simulink model "ev13_registros"  (R2023b)
settings: Solver=VariableStepAuto  StartTime=0.0  StopTime=inf  RelTol=1e-3
libraries: simulink_extras x10
settings Model: Creator=juanm  LastModifiedBy=juanm

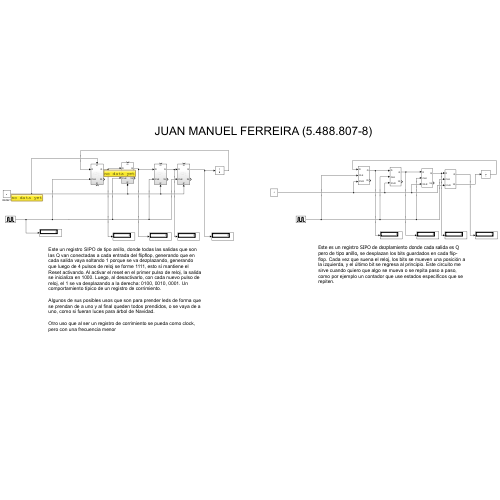
[thumbnail: Simulink's stored preview of the top-level diagram]
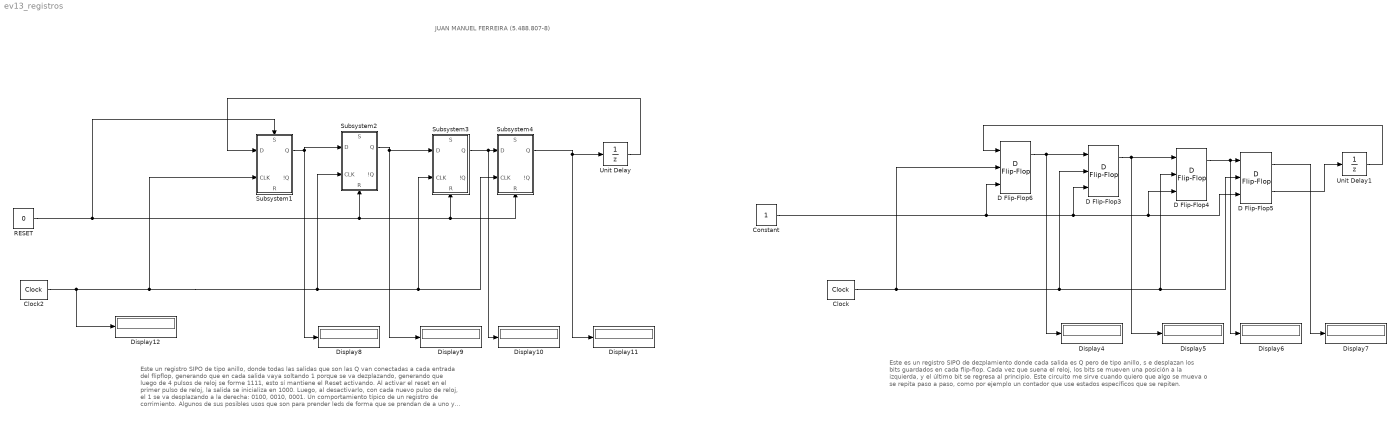
== system ev13_registros ==
  note: JUAN MANUEL FERREIRA (5.488.807-8)
  note: Este es un registro SIPO de dezplamiento donde cada salida es Q pero de tipo anillo, s e desplazan los bits guardados en cada flip-flop. Cada vez que suena el reloj, los bits se mueven una posición a la izquierda, y el último bit se regresa al principio. Este circuito me sirve cuando quiero que algo se mueva o se repita paso a paso, como por ejemplo un contador que use estados específicos que se repiten.
  note: Este un registro SIPO de tipo anillo, donde todas las salidas que son las Q van conectadas a cada entrada del flipflop, generando que en cada salida vaya soltando 1 porque se va dezplazando, generando que luego de 4 pulsos de reloj se forme 1111, esto sí mantiene el Reset activando. Al activar el reset en el primer pulso de reloj, la salida se inicializa en 1000. Luego, al desactivarlo, con cada nuevo pulso de reloj, el 1 se va desplazando a la derecha: 0100, 0010, 0001. Un comportamiento típico de un registro de corrimiento.
      |
      | Algunos de sus posibles usos que son para prender leds de forma que se prendan de a uno y al final queden todos prendidos, o se vaya de a uno, como si fueran luces para árbol de Navidad.
      |
      | Otro uso que al ser un registro de corrimiento se pueda como clock, pero con una frecuencia menor
  Clock : simulink_extras/Flip Flops/Clock  period=2
  Clock2 : simulink_extras/Flip Flops/Clock  period=2
  Constant : Constant
  D Flip-Flop{3..6} (4 alike) : simulink_extras/Flip Flops/D Flip-Flop
  Display{4..12} (9 alike) : Display
  RESET : Constant  Value=0  OutDataTypeStr=boolean
  Subsystem1 : Subsystem
      settings: PortSchema="{\"entries\":[{\"content\":{\"sides\":[{\"content\":{\"connectorIds\":[\"In1\",\"In2\"]},\"type\":\"ConnectorPlacement.EquallySpacedRectSide\",\"uuid\":\"e3878c95-46f3-4509-9baa-e715f418dba1\"},{\"content\":{\"connectorIds\":[\"Out1\",\"Out2\"],\"side\":\"RIGHT\"},\"type\":\"ConnectorPlacement.EquallySpacedRectSide\",\"uuid\":\"07877722-e247-4eb2-8428-8296816940c1\"},{\"content\":{\"connectorIds\":[\"In3\"],\"side\":\"TOP\"},\"type\":\"ConnectorPlacement.EquallySpacedRectSide\",\"uuid\":\"8cc11adc-8fe2-4fc3-91be-12b2d4a599d3\"},{\"content\":{\"connectorIds\":[\"In4\"],\"side\":\"BOTTOM\"},\"type\":\"ConnectorPlacement.EquallySpacedRectSide\",\"uuid\":\"07da6bee-c4ce-4432-ad6f-4d7b93f4049b\"}]},\"type\":\"ConnectorPlacement.EquallySpacedConnector\",\"uuid\":\"c12c8677-41de-4e24-9f13-5794546de7c9\"}],\"packageUris\":[\"http://schema.mathworks.com/mf0/Connector/R2020b\"],\"version\":\"1.0\"}"
  Subsystem2 : Subsystem
      settings: PortSchema="{\"entries\":[{\"content\":{\"sides\":[{\"content\":{\"connectorIds\":[\"In1\",\"In2\"]},\"type\":\"ConnectorPlacement.EquallySpacedRectSide\",\"uuid\":\"e3878c95-46f3-4509-9baa-e715f418dba1\"},{\"content\":{\"connectorIds\":[\"Out1\",\"Out2\"],\"side\":\"RIGHT\"},\"type\":\"ConnectorPlacement.EquallySpacedRectSide\",\"uuid\":\"07877722-e247-4eb2-8428-8296816940c1\"},{\"content\":{\"connectorIds\":[\"In3\"],\"side\":\"TOP\"},\"type\":\"ConnectorPlacement.EquallySpacedRectSide\",\"uuid\":\"8cc11adc-8fe2-4fc3-91be-12b2d4a599d3\"},{\"content\":{\"connectorIds\":[\"In4\"],\"side\":\"BOTTOM\"},\"type\":\"ConnectorPlacement.EquallySpacedRectSide\",\"uuid\":\"07da6bee-c4ce-4432-ad6f-4d7b93f4049b\"}]},\"type\":\"ConnectorPlacement.EquallySpacedConnector\",\"uuid\":\"c12c8677-41de-4e24-9f13-5794546de7c9\"}],\"packageUris\":[\"http://schema.mathworks.com/mf0/Connector/R2020b\"],\"version\":\"1.0\"}"
  Subsystem3 : Subsystem
      settings: PortSchema="{\"entries\":[{\"content\":{\"sides\":[{\"content\":{\"connectorIds\":[\"In1\",\"In2\"]},\"type\":\"ConnectorPlacement.EquallySpacedRectSide\",\"uuid\":\"e3878c95-46f3-4509-9baa-e715f418dba1\"},{\"content\":{\"connectorIds\":[\"Out1\",\"Out2\"],\"side\":\"RIGHT\"},\"type\":\"ConnectorPlacement.EquallySpacedRectSide\",\"uuid\":\"07877722-e247-4eb2-8428-8296816940c1\"},{\"content\":{\"connectorIds\":[\"In3\"],\"side\":\"TOP\"},\"type\":\"ConnectorPlacement.EquallySpacedRectSide\",\"uuid\":\"8cc11adc-8fe2-4fc3-91be-12b2d4a599d3\"},{\"content\":{\"connectorIds\":[\"In4\"],\"side\":\"BOTTOM\"},\"type\":\"ConnectorPlacement.EquallySpacedRectSide\",\"uuid\":\"07da6bee-c4ce-4432-ad6f-4d7b93f4049b\"}]},\"type\":\"ConnectorPlacement.EquallySpacedConnector\",\"uuid\":\"c12c8677-41de-4e24-9f13-5794546de7c9\"}],\"packageUris\":[\"http://schema.mathworks.com/mf0/Connector/R2020b\"],\"version\":\"1.0\"}"
  Subsystem4 : Subsystem
      settings: PortSchema="{\"entries\":[{\"content\":{\"sides\":[{\"content\":{\"connectorIds\":[\"In1\",\"In2\"]},\"type\":\"ConnectorPlacement.EquallySpacedRectSide\",\"uuid\":\"e3878c95-46f3-4509-9baa-e715f418dba1\"},{\"content\":{\"connectorIds\":[\"Out1\",\"Out2\"],\"side\":\"RIGHT\"},\"type\":\"ConnectorPlacement.EquallySpacedRectSide\",\"uuid\":\"07877722-e247-4eb2-8428-8296816940c1\"},{\"content\":{\"connectorIds\":[\"In3\"],\"side\":\"TOP\"},\"type\":\"ConnectorPlacement.EquallySpacedRectSide\",\"uuid\":\"8cc11adc-8fe2-4fc3-91be-12b2d4a599d3\"},{\"content\":{\"connectorIds\":[\"In4\"],\"side\":\"BOTTOM\"},\"type\":\"ConnectorPlacement.EquallySpacedRectSide\",\"uuid\":\"07da6bee-c4ce-4432-ad6f-4d7b93f4049b\"}]},\"type\":\"ConnectorPlacement.EquallySpacedConnector\",\"uuid\":\"c12c8677-41de-4e24-9f13-5794546de7c9\"}],\"packageUris\":[\"http://schema.mathworks.com/mf0/Connector/R2020b\"],\"version\":\"1.0\"}"
  Unit Delay : UnitDelay  SampleTime=-1  HasFrameUpgradeWarning=on
  Unit Delay1 : UnitDelay  SampleTime=-1  HasFrameUpgradeWarning=on
  wires:
  D Flip-Flop3/1 -> D Flip-Flop4/1, Display5/1
  D Flip-Flop4/1 -> D Flip-Flop5/1, Display6/1
  Unit Delay1/1 -> D Flip-Flop6/1
  D Flip-Flop6/1 -> D Flip-Flop3/1, Display4/1
  Clock/1 -> D Flip-Flop3/2, D Flip-Flop4/2, D Flip-Flop5/2, D Flip-Flop6/2
  Constant/1 -> D Flip-Flop6/3, D Flip-Flop3/3, D Flip-Flop4/3, D Flip-Flop5/3
  D Flip-Flop5/2 -> Unit Delay1/1
  D Flip-Flop5/1 -> Display7/1
  Subsystem2/1(Q) -> Subsystem3/1(D), Display9/1
  Subsystem3/1(Q) -> Subsystem4/1(D), Display10/1
  Subsystem4/1(Q) -> Display11/1, Unit Delay/1
  Subsystem1/1(Q) -> Subsystem2/1(D), Display8/1
  Clock2/1 -> Display12/1, Subsystem1/2(CLK), Subsystem2/2(CLK), Subsystem3/2(CLK), Subsystem4/2(CLK)
  RESET/1 -> Subsystem2/4(R), Subsystem3/4(R), Subsystem4/4(R), Subsystem1/3(S)
  Unit Delay/1 -> Subsystem1/1(D)

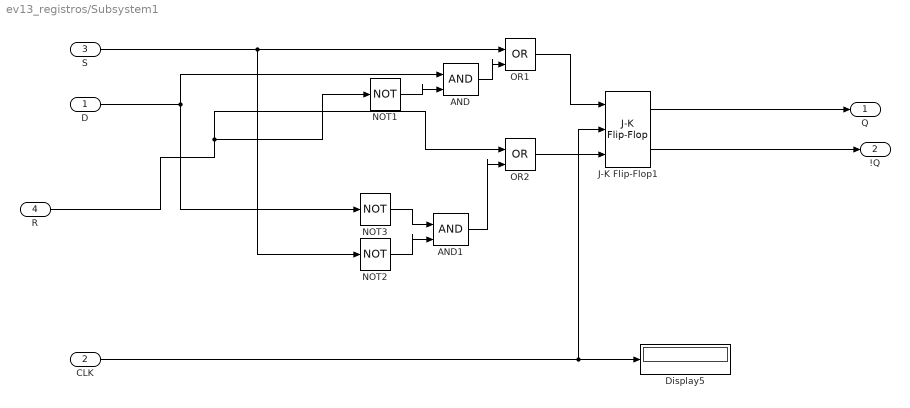
== system ev13_registros/Subsystem1 ==
  D : Inport
  CLK : Inport  Port=2
  S : Inport  Port=3
  R : Inport  Port=4
  AND : Logic  IconShape=distinctive  AllPortsSameDT=off  OutDataTypeStr=boolean
  AND1 : Logic  IconShape=distinctive  AllPortsSameDT=off  OutDataTypeStr=boolean
  Display5 : Display
  J-K Flip-Flop1 : simulink_extras/Flip Flops/J-K Flip-Flop  initial_condition=0
  NOT1 : Logic  Operator=NOT  IconShape=distinctive  AllPortsSameDT=off  OutDataTypeStr=boolean
  NOT2 : Logic  Operator=NOT  IconShape=distinctive  AllPortsSameDT=off  OutDataTypeStr=boolean
  NOT3 : Logic  Operator=NOT  IconShape=distinctive  AllPortsSameDT=off  OutDataTypeStr=boolean
  OR1 : Logic  Operator=OR  IconShape=distinctive  AllPortsSameDT=off  OutDataTypeStr=boolean
  OR2 : Logic  Operator=OR  IconShape=distinctive  AllPortsSameDT=off  OutDataTypeStr=boolean
  Q : Outport
  !Q : Outport  Port=2
  wires:
  R/1 -> NOT1/1, OR2/1
  S/1 -> OR1/1, NOT2/1
  J-K Flip-Flop1/1 -> Q/1
  AND/1 -> OR1/2
  NOT2/1 -> AND1/2
  NOT1/1 -> AND/2
  OR2/1 -> J-K Flip-Flop1/3
  CLK/1 -> Display5/1, J-K Flip-Flop1/2
  AND1/1 -> OR2/2
  J-K Flip-Flop1/2 -> !Q/1
  OR1/1 -> J-K Flip-Flop1/1
  NOT3/1 -> AND1/1
  D/1 -> AND/1, NOT3/1

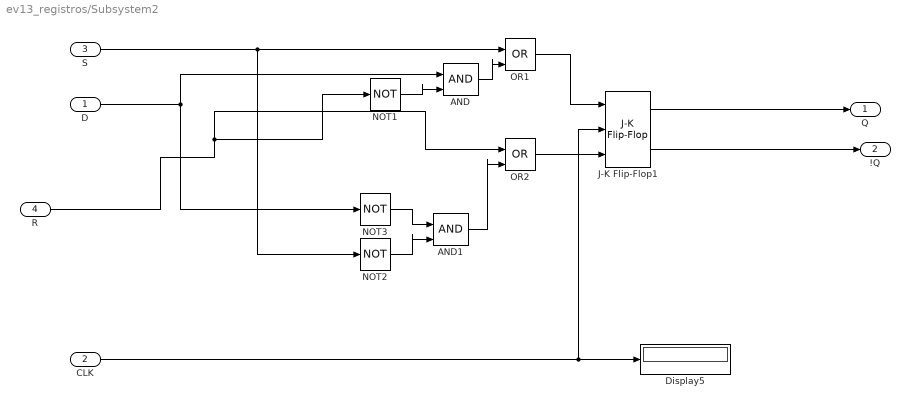
== system ev13_registros/Subsystem2 ==
  D : Inport
  CLK : Inport  Port=2
  S : Inport  Port=3
  R : Inport  Port=4
  AND : Logic  IconShape=distinctive  AllPortsSameDT=off  OutDataTypeStr=boolean
  AND1 : Logic  IconShape=distinctive  AllPortsSameDT=off  OutDataTypeStr=boolean
  Display5 : Display
  J-K Flip-Flop1 : simulink_extras/Flip Flops/J-K Flip-Flop  initial_condition=0
  NOT1 : Logic  Operator=NOT  IconShape=distinctive  AllPortsSameDT=off  OutDataTypeStr=boolean
  NOT2 : Logic  Operator=NOT  IconShape=distinctive  AllPortsSameDT=off  OutDataTypeStr=boolean
  NOT3 : Logic  Operator=NOT  IconShape=distinctive  AllPortsSameDT=off  OutDataTypeStr=boolean
  OR1 : Logic  Operator=OR  IconShape=distinctive  AllPortsSameDT=off  OutDataTypeStr=boolean
  OR2 : Logic  Operator=OR  IconShape=distinctive  AllPortsSameDT=off  OutDataTypeStr=boolean
  Q : Outport
  !Q : Outport  Port=2
  wires:
  D/1 -> NOT3/1, AND/1
  NOT3/1 -> AND1/1
  OR1/1 -> J-K Flip-Flop1/1
  J-K Flip-Flop1/2 -> !Q/1
  AND1/1 -> OR2/2
  CLK/1 -> J-K Flip-Flop1/2, Display5/1
  OR2/1 -> J-K Flip-Flop1/3
  NOT1/1 -> AND/2
  NOT2/1 -> AND1/2
  AND/1 -> OR1/2
  J-K Flip-Flop1/1 -> Q/1
  S/1 -> NOT2/1, OR1/1
  R/1 -> OR2/1, NOT1/1

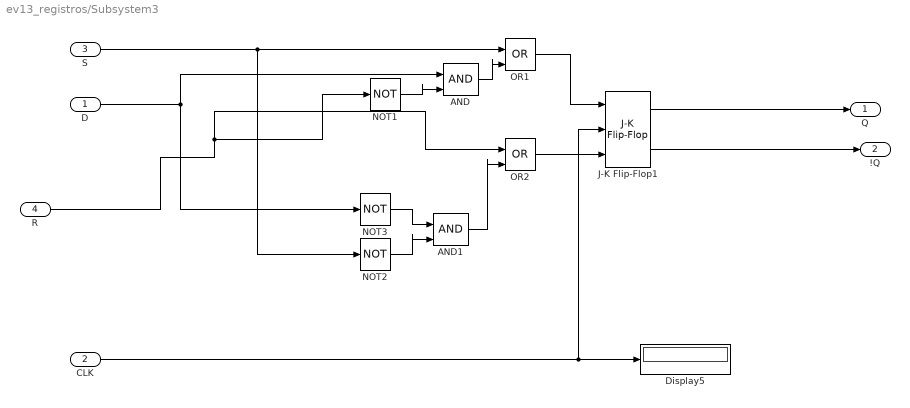
== system ev13_registros/Subsystem3 ==
  D : Inport
  CLK : Inport  Port=2
  S : Inport  Port=3
  R : Inport  Port=4
  AND : Logic  IconShape=distinctive  AllPortsSameDT=off  OutDataTypeStr=boolean
  AND1 : Logic  IconShape=distinctive  AllPortsSameDT=off  OutDataTypeStr=boolean
  Display5 : Display
  J-K Flip-Flop1 : simulink_extras/Flip Flops/J-K Flip-Flop  initial_condition=0
  NOT1 : Logic  Operator=NOT  IconShape=distinctive  AllPortsSameDT=off  OutDataTypeStr=boolean
  NOT2 : Logic  Operator=NOT  IconShape=distinctive  AllPortsSameDT=off  OutDataTypeStr=boolean
  NOT3 : Logic  Operator=NOT  IconShape=distinctive  AllPortsSameDT=off  OutDataTypeStr=boolean
  OR1 : Logic  Operator=OR  IconShape=distinctive  AllPortsSameDT=off  OutDataTypeStr=boolean
  OR2 : Logic  Operator=OR  IconShape=distinctive  AllPortsSameDT=off  OutDataTypeStr=boolean
  Q : Outport
  !Q : Outport  Port=2
  wires:
  R/1 -> NOT1/1, OR2/1
  S/1 -> OR1/1, NOT2/1
  J-K Flip-Flop1/1 -> Q/1
  AND/1 -> OR1/2
  NOT2/1 -> AND1/2
  NOT1/1 -> AND/2
  OR2/1 -> J-K Flip-Flop1/3
  CLK/1 -> Display5/1, J-K Flip-Flop1/2
  AND1/1 -> OR2/2
  J-K Flip-Flop1/2 -> !Q/1
  OR1/1 -> J-K Flip-Flop1/1
  NOT3/1 -> AND1/1
  D/1 -> AND/1, NOT3/1

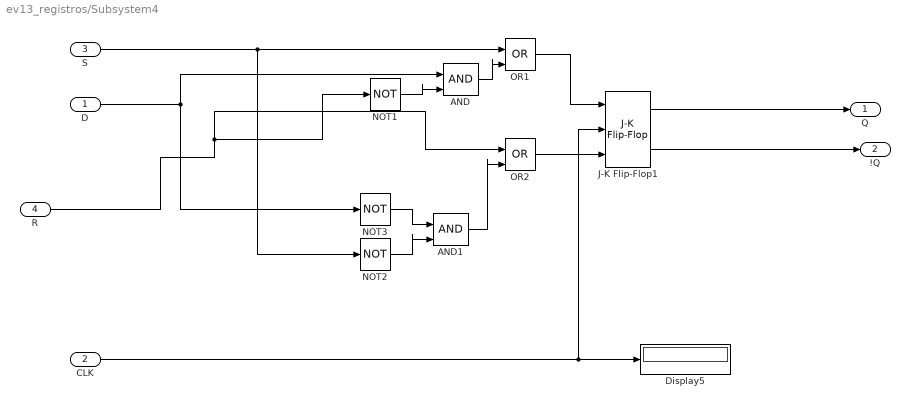
== system ev13_registros/Subsystem4 ==
  D : Inport
  CLK : Inport  Port=2
  S : Inport  Port=3
  R : Inport  Port=4
  AND : Logic  IconShape=distinctive  AllPortsSameDT=off  OutDataTypeStr=boolean
  AND1 : Logic  IconShape=distinctive  AllPortsSameDT=off  OutDataTypeStr=boolean
  Display5 : Display
  J-K Flip-Flop1 : simulink_extras/Flip Flops/J-K Flip-Flop  initial_condition=0
  NOT1 : Logic  Operator=NOT  IconShape=distinctive  AllPortsSameDT=off  OutDataTypeStr=boolean
  NOT2 : Logic  Operator=NOT  IconShape=distinctive  AllPortsSameDT=off  OutDataTypeStr=boolean
  NOT3 : Logic  Operator=NOT  IconShape=distinctive  AllPortsSameDT=off  OutDataTypeStr=boolean
  OR1 : Logic  Operator=OR  IconShape=distinctive  AllPortsSameDT=off  OutDataTypeStr=boolean
  OR2 : Logic  Operator=OR  IconShape=distinctive  AllPortsSameDT=off  OutDataTypeStr=boolean
  Q : Outport
  !Q : Outport  Port=2
  wires:
  D/1 -> NOT3/1, AND/1
  NOT3/1 -> AND1/1
  OR1/1 -> J-K Flip-Flop1/1
  J-K Flip-Flop1/2 -> !Q/1
  AND1/1 -> OR2/2
  CLK/1 -> J-K Flip-Flop1/2, Display5/1
  OR2/1 -> J-K Flip-Flop1/3
  NOT1/1 -> AND/2
  NOT2/1 -> AND1/2
  AND/1 -> OR1/2
  J-K Flip-Flop1/1 -> Q/1
  S/1 -> NOT2/1, OR1/1
  R/1 -> OR2/1, NOT1/1
